simulink model "fridge"  (R2026a)
settings: Solver=VariableStepAuto
settings Model: Creator=tovi  LastModifiedBy=tdxt

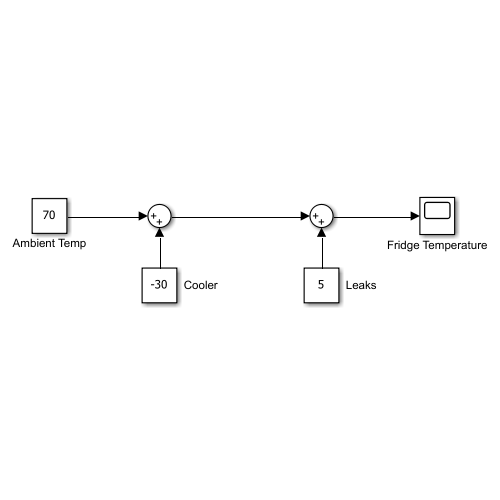
[thumbnail: Simulink's stored preview of the top-level diagram]
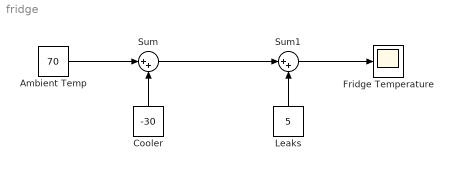
== system fridge ==
  Ambient Temp : Constant  Value=70
  Cooler : Constant  Value=-30
  Fridge Temperature : Scope
      settings: ActiveDisplayYMinimum=28.502859274714829  ActiveDisplayYMaximum=62.70964643704113
  Leaks : Constant  Value=5
  Sum : Sum  Inputs=|++
  Sum1 : Sum  Inputs=|++
  wires:
  Ambient Temp/1 -> Sum/1
  Cooler/1 -> Sum/2
  Sum/1 -> Sum1/1
  Sum1/1 -> Fridge Temperature/1
  Leaks/1 -> Sum1/2
